simulink model "Sub_sys_4_varying_Rs"  (R2024a)
settings: Solver=ode45  StartTime=0.0  StopTime=4  MaxStep=0.02  RelTol=1e-3  EnableMultiTasking=on
libraries: simulink x2
settings Model: Creator=motahhir  LastModifiedBy=Aswathi Sajeev
settings SolverCC: AlgebraicLoopSolver=TrustRegion
settings DataIOCC: LimitDataPoints=on  SaveFormat=Array  SignalLoggingSaveFormat=ModelDataLogs  ReturnWorkspaceOutputs=off
settings OptimizationCC: ExpressionDepthLimit=2147483647  LifeSpan=inf
settings DebuggingCC: UnderspecifiedInitializationDetection=Classic  MergeDetectMultiDrivingBlocksExec=none  SolverPrmCheckMsg=warning  FcnCallInpInsideContextMsg=warning  UnconnectedInputMsg=warning  UnconnectedOutputMsg=warning  UnconnectedLineMsg=warning  StateNameClashWarn=warning  SFUnexpectedBacktrackingDiag=warning  SFNoUnconditionalDefaultTransitionDiag=warning  ArithmeticOperatorsInVariantConditions=warning
settings HardwareCC: ProdBitPerPointer=32  ProdBitPerSizeT=32  ProdBitPerPtrDiffT=32  ProdLargestAtomicFloat=None  ProdIntDivRoundTo=Undefined  ProdEndianess=Unspecified  ProdWordSize=32  ProdHWDeviceType=32-bit Generic
settings ModelReferenceCC: EnableRefExpFcnMdlSchedulingChecks=on  PropagateSignalLabelsOutOfModel=off
settings SFSimCC: SimUseLocalCustomCode=off  CustomCodeUndefinedFunction=UseInterfaceOnly
settings RTWCC: RTWUseLocalCustomCode=off  GPUComputeCapability=3.5
settings CodeAppCC: StateflowObjectComments=on
settings GRTTargetCC: TargetLangStandard=C89/C90 (ANSI)
settings ConfigComp: CovMetricSettings=dw  CovSaveCumulativeToWorkspaceVar=on  CovSaveSingleToWorkspaceVar=on  CovExternalEMLEnable=off  CovSFcnEnable=off

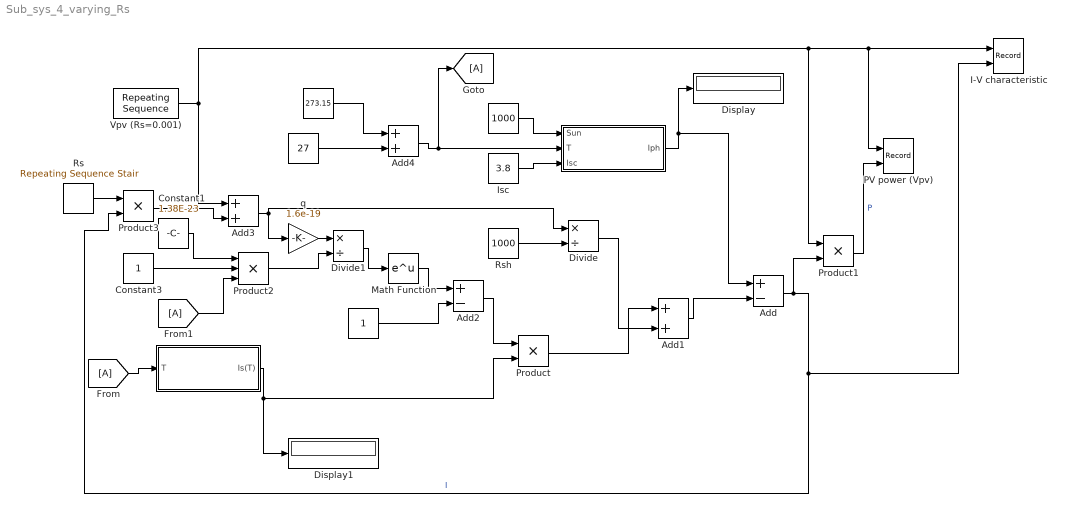
== system Sub_sys_4_varying_Rs ==
  "  " : Constant  Value=27
  "   " : Subsystem
  "    " : Constant  Value=273.15
  "     " : Subsystem
      mask init:
      | q=1.6e-19;
      | T=300.15;
      | Tnom=300.15;
      | K=1.38e-23;
      | N=1.5;
      | vt=T*K/q;
      | Is=1e-9;
      | Eg=1.12;
  "                      " : Constant
  " " : Constant  Value=1000
  Add : Sum  Inputs=+-
  Add1 : Sum
  Add2 : Sum  Inputs=+-
  Add3 : Sum
  Add4 : Sum
  Constant1 : Constant  Value=1.38E-23
  Constant3 : Constant
  Display : Display
  Display1 : Display
  Divide : Product  Inputs=*/
  Divide1 : Product  Inputs=*/
  From : From
  From1 : From
  Goto : Goto
  I-V characteristic : Record  FileSettingsInternal="{\"entries\":[{\"content\":{\"excelSettings\":{\"content\":{},\"type\":\"Streamout.ExcelSettings\"}},\"type\":\"Streamout.FileSettingStorage\",\"uuid\":\"\"}],\"packageUris\":[\"http:\\/\\/schema.mathworks.com\\/mf0\\/streamout_blocks\\/R2020a\"],\"version\":\"1.0\"}"  Layout=[1 1]  SignalsInternal="{\"entries\":[{\"content\":{\"signals\":[{\"content\":{\"blockPath\":[],\"dimensions\":[1],\"domain\":\"\",\"lineColor\":\"#22b573\",\"plots\":[ 1 ],\"port\":1,\"sid\":[\"\"],\"signalID\":1,\"signalName\":\"Vpv (Rs=0.001)\"},\"type\":\"RecordBlkView.Signal\",\"uuid\":\"\"},{\"content\":{\"blockPath\":[],\"dimensions\":[1],\"domain\":\"\",\"lineColor\":\"#22b573\",\"plots\":[ 1 ],\"port\":2,\"sid\":[\"\"],\"signalID\":2,\"signalName\":\"I\"},\"type\":\"RecordBlkView.Signal\",\"uuid\":\"\"}]},\"type\":\"RecordBlkView.InputSignals\",\"uuid\":\"\"}],\"packageUris\":[\"http:\\/\\/schema.mathworks.com\\/mf0\\/streamout_blocks\\/R2020a\"],\"version\":\"1.0\"}"  VisualizationBindings="{\"xyplotplugin\":{\"info\":[{\"series\":[{\"bindingParametersList\":[{\"parameter\":\"X-Axis\",\"signalID\":1,\"signalName\":\"Vpv (Rs=0.001)\"},{\"parameter\":\"Y-Axis\",\"signalID\":2,\"signalName\":\"I\"}],\"seriesID\":0}],\"subplotID\":1}]}}"  CompatibilityTag=XY  st=-1
  Isc : Constant  Value=3.8
  Math Function : Math  SignedPower=on
  PV power (Vpv) : Record  FileSettingsInternal="{\"entries\":[{\"content\":{\"excelSettings\":{\"content\":{},\"type\":\"Streamout.ExcelSettings\"}},\"type\":\"Streamout.FileSettingStorage\",\"uuid\":\"\"}],\"packageUris\":[\"http:\\/\\/schema.mathworks.com\\/mf0\\/streamout_blocks\\/R2020a\"],\"version\":\"1.0\"}"  Layout=[1 1]  SignalsInternal="{\"entries\":[{\"content\":{\"signals\":[{\"content\":{\"blockPath\":[],\"dimensions\":[1],\"domain\":\"\",\"lineColor\":\"#77ac30\",\"plots\":[ 1 ],\"port\":1,\"sid\":[\"\"],\"signalID\":1,\"signalName\":\"Vpv (Rs=0.001)\"},\"type\":\"RecordBlkView.Signal\",\"uuid\":\"\"},{\"content\":{\"blockPath\":[],\"dimensions\":[1],\"domain\":\"\",\"lineColor\":\"#77ac30\",\"plots\":[ 1 ],\"port\":2,\"sid\":[\"\"],\"signalID\":2,\"signalName\":\"P\"},\"type\":\"RecordBlkView.Signal\",\"uuid\":\"\"}]},\"type\":\"RecordBlkView.InputSignals\",\"uuid\":\"\"}],\"packageUris\":[\"http:\\/\\/schema.mathworks.com\\/mf0\\/streamout_blocks\\/R2020a\"],\"version\":\"1.0\"}"  VisualizationBindings="{\"xyplotplugin\":{\"info\":[{\"series\":[{\"bindingParametersList\":[{\"parameter\":\"X-Axis\",\"signalID\":1,\"signalName\":\"Vpv (Rs=0.001)\"},{\"parameter\":\"Y-Axis\",\"signalID\":2,\"signalName\":\"P\"}],\"seriesID\":0}],\"subplotID\":1}]}}"  CompatibilityTag=XY  st=-1
  Product : Product  RndMeth=Zero
  Product1 : Product  RndMeth=Zero
  Product2 : Product  Inputs=3  RndMeth=Zero
  Product3 : Product  RndMeth=Zero
  Rs : simulink/Sources/Repeating Sequence Stair  OutValues=[0.001].'  tsamp=1  OutMin=[]  OutMax=[]  OutDataTypeStr=float('double')  OutputDataTypeScalingMode=Specify via dialog  OutDataType=float('double')  ConRadixGroup=Best Precision: Vector-wise  OutScaling=2^-12
  Rsh : Constant  Value=1000
  Vpv (Rs=0.001) : simulink/Sources/Repeating Sequence  rep_seq_t=[0 1 2]  rep_seq_y="[-0.1  0.6 -0.1]"
  q : Gain  Gain=1.6e-19
  wires:
  Isc/1 -> "   "/3(Isc)
  Add4/1 -> "   "/2(T), Goto/1
  "   "/1(Iph) -> Display/1, Add/1
  From/1 -> "     "/1(T)
  Divide/1 -> Add1/2
  Rsh/1 -> Divide/2
  "     "/1(Is(T)) -> Product/2, Display1/1
  Add2/1 -> Product/1
  Math Function/1 -> Add2/1
  "                      "/1 -> Add2/2
  Divide1/1 -> Math Function/1
  Add/1 -> Product1/2, I-V characteristic/2, Product3/2  "I"
  Product1/1 -> PV power (Vpv)/2  "P"
  Product/1 -> Add1/1
  Add1/1 -> Add/2
  Vpv (Rs=0.001)/1 -> Add3/1, PV power (Vpv)/1, I-V characteristic/1, Product1/1
  q/1 -> Divide1/1
  Add3/1 -> q/1, Divide/1
  Constant1/1 -> Product2/1
  From1/1 -> Product2/3
  Constant3/1 -> Product2/2
  Product2/1 -> Divide1/2
  "  "/1 -> Add4/2
  " "/1 -> "   "/1(Sun)
  "    "/1 -> Add4/1
  Product3/1 -> Add3/2
  Rs/1 -> Product3/1

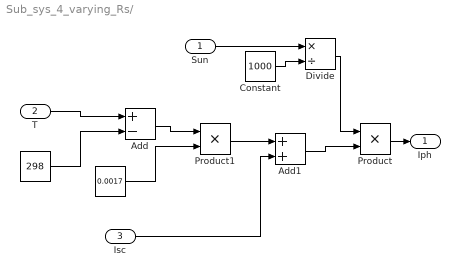
== system Sub_sys_4_varying_Rs/    ==
  Sun : Inport
  T : Inport  Port=2
  Isc : Inport  Port=3
  "  " : Constant  Value=0.0017
  "   " : Constant  Value=298
  Add : Sum  Inputs=+-
  Add1 : Sum
  Constant : Constant  Value=1000
  Divide : Product  Inputs=*/
  Product : Product  RndMeth=Zero
  Product1 : Product  RndMeth=Zero
  Iph : Outport
  wires:
  Product/1 -> Iph/1
  Sun/1 -> Divide/1
  Constant/1 -> Divide/2
  T/1 -> Add/1
  "   "/1 -> Add/2
  Add/1 -> Product1/1
  "  "/1 -> Product1/2
  Product1/1 -> Add1/1
  Add1/1 -> Product/2
  Isc/1 -> Add1/2
  Divide/1 -> Product/1

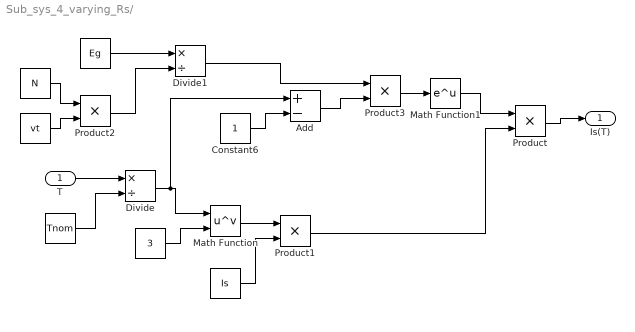
== system Sub_sys_4_varying_Rs/      ==
  T : Inport
  "  " : Constant  Value=3
  "      " : Constant  Value=Is
  "        " : Constant  Value=Tnom
  "                      " : Constant  Value=Eg
  "                              " : Constant  Value=N
  "                               " : Constant  Value=vt
  Add : Sum  Inputs=+-
  Constant6 : Constant
  Divide : Product  Inputs=*/
  Divide1 : Product  Inputs=*/
  Math Function : Math  Operator=pow  SignedPower=on
  Math Function1 : Math  SignedPower=on
  Product{,1..3} (4 alike) : Product  RndMeth=Zero
  Is(T) : Outport
  wires:
  Product/1 -> Is(T)/1
  T/1 -> Divide/1
  "        "/1 -> Divide/2
  Divide/1 -> Math Function/1, Add/1
  "  "/1 -> Math Function/2
  Math Function/1 -> Product1/1
  "      "/1 -> Product1/2
  Product1/1 -> Product/2
  "                               "/1 -> Product2/2
  "                              "/1 -> Product2/1
  Product2/1 -> Divide1/2
  "                      "/1 -> Divide1/1
  Math Function1/1 -> Product/1
  Product3/1 -> Math Function1/1
  Divide1/1 -> Product3/1
  Add/1 -> Product3/2
  Constant6/1 -> Add/2
